simulink model "TestCase2_system_mapping"  (R2016a)
settings: Solver=FixedStepAuto  StartTime=0.0  StopTime=10.0  RelTol=1e-3
model workspace: external: MAT-File TestCase2_system_mapping.mat (data not in the file)
undefined symbols (not defined in the file or in its folder): obstacle
libraries: libTLAsserts x6, libAsserts x2
settings Model: Creator=Josef  LastModifiedBy=Josef
settings HardwareCC: ProdBitPerPointer=32  ProdWordSize=32  ProdHWDeviceType=Intel->x86-32 (Windows32)
settings GRTTargetCC: GeneratePreprocessorConditionals=Use local settings

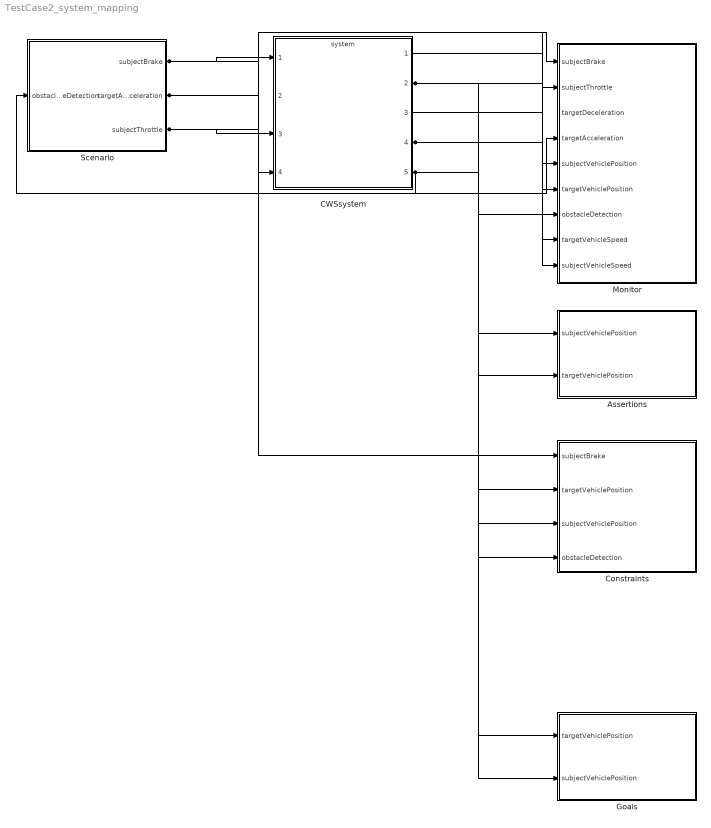
== system TestCase2_system_mapping ==
  Assertions : Subsystem
  CWSsystem : ModelReference  ModelNameDialog=system  SimulationMode=Normal  ModelReferenceVersion=1.18
  Constraints : Subsystem
  Goals : Subsystem
  Monitor : Subsystem
  Scenario : Subsystem
  wires:
  Scenario/3(subjectThrottle) -> CWSsystem/3, Monitor/2(subjectThrottle)
  Scenario/1(subjectBrake) -> CWSsystem/1, Monitor/1(subjectBrake), Constraints/1(subjectBrake)
  Scenario/2(targetAcceleration) -> CWSsystem/4, Monitor/4(targetAcceleration)
  CWSsystem/5 -> Scenario/1(obstacleDetection), Monitor/7(obstacleDetection), Constraints/4(obstacleDetection)
  CWSsystem/2 -> Monitor/5(subjectVehiclePosition), Assertions/1(subjectVehiclePosition), Constraints/3(subjectVehiclePosition), Goals/2(subjectVehiclePosition)
  CWSsystem/4 -> Monitor/6(targetVehiclePosition), Assertions/2(targetVehiclePosition), Constraints/2(targetVehiclePosition), Goals/1(targetVehiclePosition)
  CWSsystem/3 -> Monitor/8(targetVehicleSpeed)
  CWSsystem/1 -> Monitor/9(subjectVehicleSpeed)

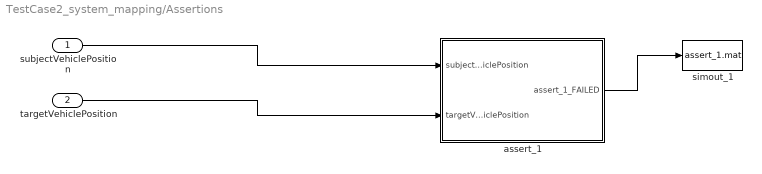
== system TestCase2_system_mapping/Assertions ==
  subjectVehiclePosition : Inport
  targetVehiclePosition : Inport  Port=2
  assert_1 : Subsystem
  simout_1 : ToFile  Filename=assert_1.mat  MatrixName=assert_1  SaveFormat=Timeseries
  wires:
  subjectVehiclePosition/1 -> assert_1/1(subjectVehiclePosition)
  targetVehiclePosition/1 -> assert_1/2(targetVehiclePosition)
  assert_1/1(assert_1_FAILED) -> simout_1/1

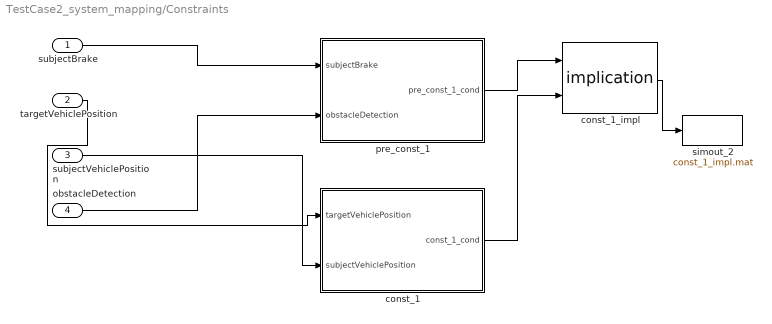
== system TestCase2_system_mapping/Constraints ==
  subjectBrake : Inport
  targetVehiclePosition : Inport  Port=2
  subjectVehiclePosition : Inport  Port=3
  obstacleDetection : Inport  Port=4
  const_1 : Subsystem
  const_1_impl : libAsserts/implication
  pre_const_1 : Subsystem
  simout_2 : ToFile  Filename=const_1_impl.mat  MatrixName=const_1_impl  SaveFormat=Timeseries
  wires:
  subjectBrake/1 -> pre_const_1/1(subjectBrake)
  obstacleDetection/1 -> pre_const_1/2(obstacleDetection)
  targetVehiclePosition/1 -> const_1/1(targetVehiclePosition)
  subjectVehiclePosition/1 -> const_1/2(subjectVehiclePosition)
  pre_const_1/1(pre_const_1_cond) -> const_1_impl/1
  const_1/1(const_1_cond) -> const_1_impl/2
  const_1_impl/1 -> simout_2/1

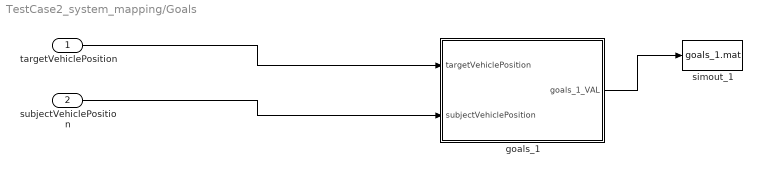
== system TestCase2_system_mapping/Goals ==
  targetVehiclePosition : Inport
  subjectVehiclePosition : Inport  Port=2
  goals_1 : Subsystem
  simout_1 : ToFile  Filename=goals_1.mat  MatrixName=goals_1  SaveFormat=Timeseries
  wires:
  targetVehiclePosition/1 -> goals_1/1(targetVehiclePosition)
  subjectVehiclePosition/1 -> goals_1/2(subjectVehiclePosition)
  goals_1/1(goals_1_VAL) -> simout_1/1

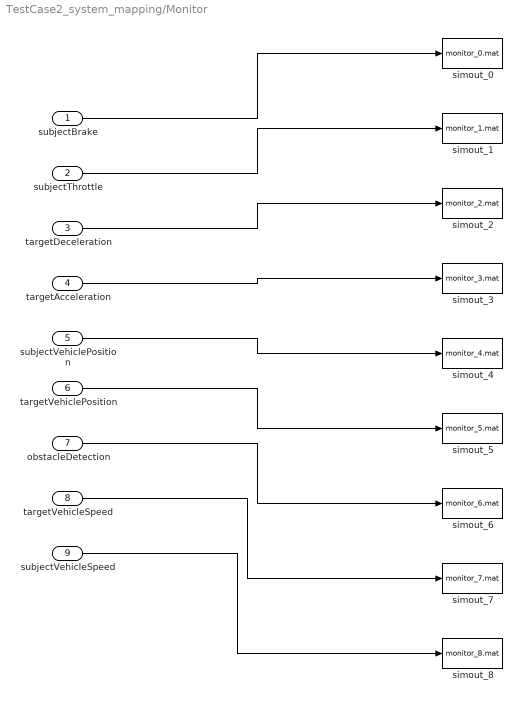
== system TestCase2_system_mapping/Monitor ==
  subjectBrake : Inport
  subjectThrottle : Inport  Port=2
  targetDeceleration : Inport  Port=3
  targetAcceleration : Inport  Port=4
  subjectVehiclePosition : Inport  Port=5
  targetVehiclePosition : Inport  Port=6
  obstacleDetection : Inport  Port=7
  targetVehicleSpeed : Inport  Port=8
  subjectVehicleSpeed : Inport  Port=9
  simout_0 : ToFile  Filename=monitor_0.mat  MatrixName=subjectBrake  SaveFormat=Timeseries
  simout_1 : ToFile  Filename=monitor_1.mat  MatrixName=subjectThrottle  SaveFormat=Timeseries
  simout_2 : ToFile  Filename=monitor_2.mat  MatrixName=targetDeceleration  SaveFormat=Timeseries
  simout_3 : ToFile  Filename=monitor_3.mat  MatrixName=targetAcceleration  SaveFormat=Timeseries
  simout_4 : ToFile  Filename=monitor_4.mat  MatrixName=subjectVehiclePosition  SaveFormat=Timeseries
  simout_5 : ToFile  Filename=monitor_5.mat  MatrixName=targetVehiclePosition  SaveFormat=Timeseries
  simout_6 : ToFile  Filename=monitor_6.mat  MatrixName=obstacleDetection  SaveFormat=Timeseries
  simout_7 : ToFile  Filename=monitor_7.mat  MatrixName=targetVehicleSpeed  SaveFormat=Timeseries
  simout_8 : ToFile  Filename=monitor_8.mat  MatrixName=subjectVehicleSpeed  SaveFormat=Timeseries
  wires:
  subjectBrake/1 -> simout_0/1
  subjectThrottle/1 -> simout_1/1
  targetDeceleration/1 -> simout_2/1
  targetAcceleration/1 -> simout_3/1
  subjectVehiclePosition/1 -> simout_4/1
  targetVehiclePosition/1 -> simout_5/1
  obstacleDetection/1 -> simout_6/1
  targetVehicleSpeed/1 -> simout_7/1
  subjectVehicleSpeed/1 -> simout_8/1

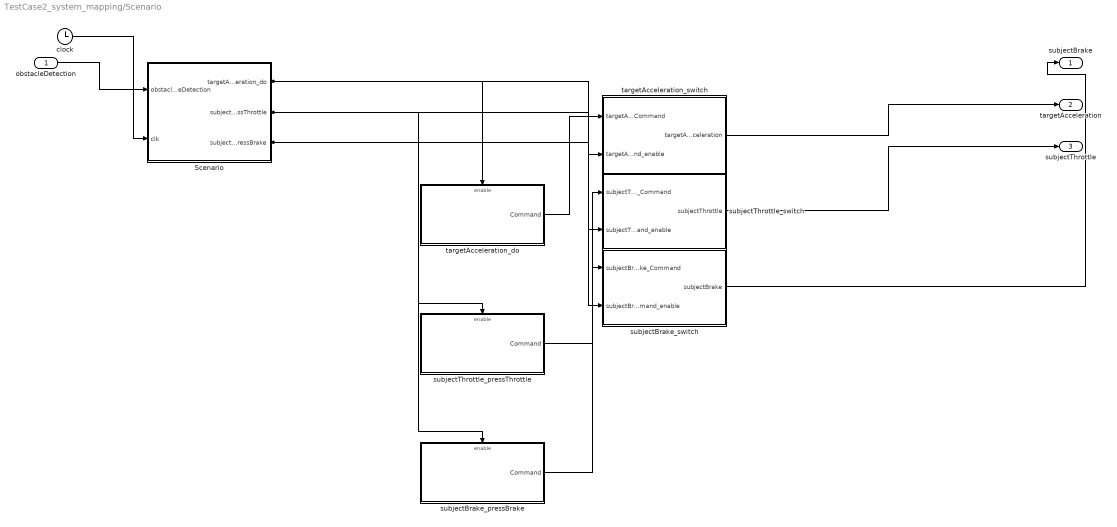
== system TestCase2_system_mapping/Scenario ==
  obstacleDetection : Inport
  Scenario : Stateflow chart  TreatAsAtomicUnit=on
  clock : Clock
  subjectBrake_pressBrake : Subsystem
  subjectBrake_switch : Subsystem
  subjectThrottle_pressThrottle : Subsystem
  subjectThrottle_switch : Subsystem
  targetAcceleration_do : Subsystem
  targetAcceleration_switch : Subsystem
  subjectBrake : Outport
  targetAcceleration : Outport  Port=2
  subjectThrottle : Outport  Port=3
  wires:
  targetAcceleration_switch/1(targetAcceleration) -> targetAcceleration/1
  subjectThrottle_switch/1(subjectThrottle) -> subjectThrottle/1
  subjectBrake_switch/1(subjectBrake) -> subjectBrake/1
  targetAcceleration_do/1(Command) -> targetAcceleration_switch/1(targetAcceleration_do_Command)
  Scenario/1(targetAcceleration_do) -> targetAcceleration_switch/2(targetAcceleration_do_Command_enable), targetAcceleration_do/Enable
  subjectThrottle_pressThrottle/1(Command) -> subjectThrottle_switch/1(subjectThrottle_pressThrottle_Command)
  Scenario/2(subjectThrottle_pressThrottle) -> subjectThrottle_switch/2(subjectThrottle_pressThrottle_Command_enable), subjectThrottle_pressThrottle/Enable
  subjectBrake_pressBrake/1(Command) -> subjectBrake_switch/1(subjectBrake_pressBrake_Command)
  Scenario/3(subjectBrake_pressBrake) -> subjectBrake_switch/2(subjectBrake_pressBrake_Command_enable), subjectBrake_pressBrake/Enable
  obstacleDetection/1 -> Scenario/1(obstacleDetection)
  clock/1 -> Scenario/2(clk)

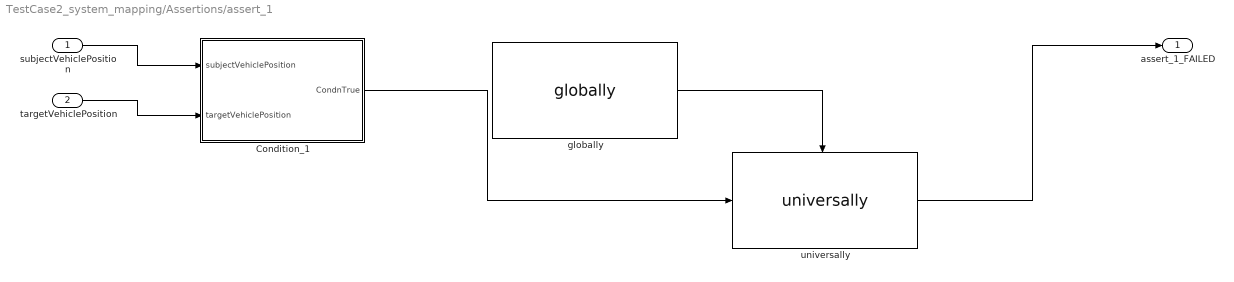
== system TestCase2_system_mapping/Assertions/assert_1 ==
  subjectVehiclePosition : Inport
  targetVehiclePosition : Inport  Port=2
  Condition_1 : Subsystem
  globally : libTLAsserts/globally
  universally : libTLAsserts/universally
  assert_1_FAILED : Outport
  wires:
  subjectVehiclePosition/1 -> Condition_1/1(subjectVehiclePosition)
  targetVehiclePosition/1 -> Condition_1/2(targetVehiclePosition)
  Condition_1/1(CondnTrue) -> universally/1
  globally/1 -> universally/Enable
  universally/1 -> assert_1_FAILED/1

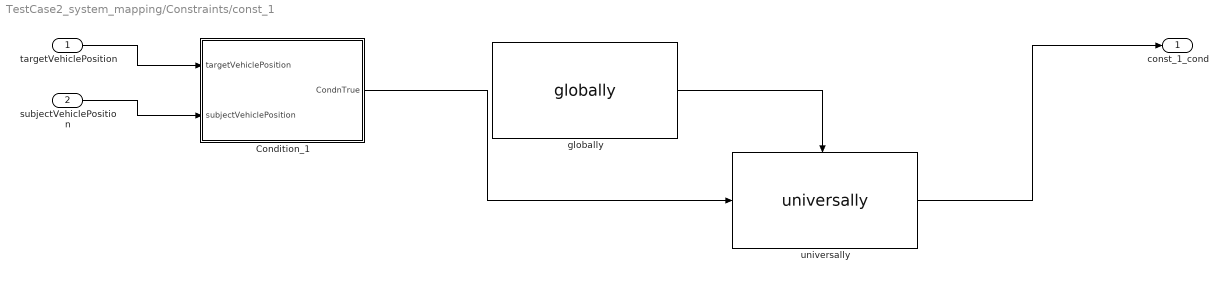
== system TestCase2_system_mapping/Constraints/const_1 ==
  targetVehiclePosition : Inport
  subjectVehiclePosition : Inport  Port=2
  Condition_1 : Subsystem
  globally : libTLAsserts/globally
  universally : libTLAsserts/universally
  const_1_cond : Outport
  wires:
  targetVehiclePosition/1 -> Condition_1/1(targetVehiclePosition)
  subjectVehiclePosition/1 -> Condition_1/2(subjectVehiclePosition)
  Condition_1/1(CondnTrue) -> universally/1
  globally/1 -> universally/Enable
  universally/1 -> const_1_cond/1

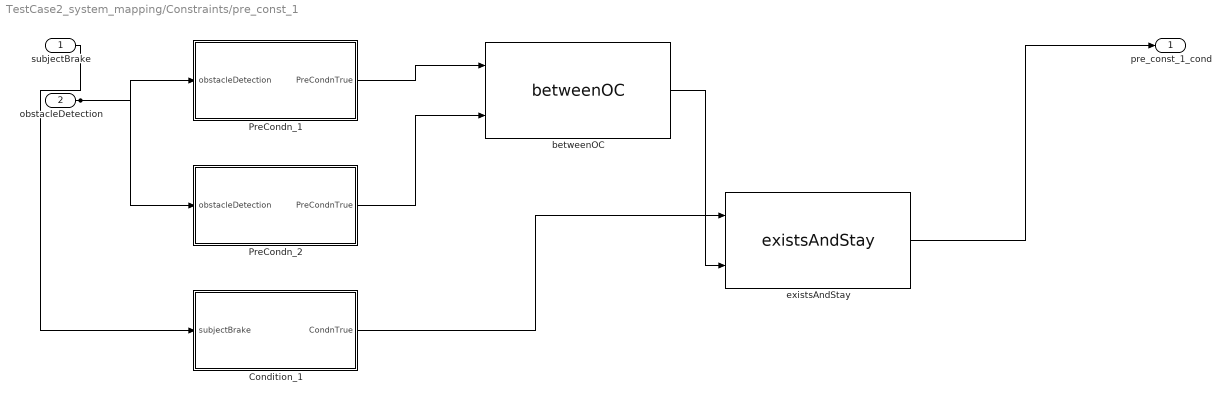
== system TestCase2_system_mapping/Constraints/pre_const_1 ==
  subjectBrake : Inport
  obstacleDetection : Inport  Port=2
  Condition_1 : Subsystem
  PreCondn_1 : Subsystem
  PreCondn_2 : Subsystem
  betweenOC : libTLAsserts/betweenOC
  existsAndStay : libTLAsserts/existsAndStay
  pre_const_1_cond : Outport
  wires:
  obstacleDetection/1 -> PreCondn_1/1(obstacleDetection), PreCondn_2/1(obstacleDetection)
  subjectBrake/1 -> Condition_1/1(subjectBrake)
  PreCondn_1/1(PreCondnTrue) -> betweenOC/1
  PreCondn_2/1(PreCondnTrue) -> betweenOC/2
  Condition_1/1(CondnTrue) -> existsAndStay/1
  betweenOC/1 -> existsAndStay/2
  existsAndStay/1 -> pre_const_1_cond/1

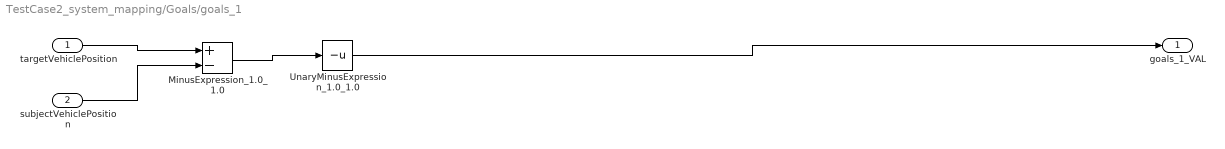
== system TestCase2_system_mapping/Goals/goals_1 ==
  targetVehiclePosition : Inport
  subjectVehiclePosition : Inport  Port=2
  MinusExpression_1.0_1.0 : Sum  Inputs=+-
  UnaryMinusExpression_1.0_1.0 : UnaryMinus
  goals_1_VAL : Outport
  wires:
  targetVehiclePosition/1 -> MinusExpression_1.0_1.0/1
  subjectVehiclePosition/1 -> MinusExpression_1.0_1.0/2
  MinusExpression_1.0_1.0/1 -> UnaryMinusExpression_1.0_1.0/1
  UnaryMinusExpression_1.0_1.0/1 -> goals_1_VAL/1

== system TestCase2_system_mapping/Scenario/subjectBrake_pressBrake ==
  Enable : EnablePort
  PedalPressed : Constant
  Command : Outport  OutputWhenDisabled=reset  InitialOutput=0
  wires:
  PedalPressed/1 -> Command/1

== system TestCase2_system_mapping/Scenario/subjectBrake_switch ==
  subjectBrake_pressBrake_Command : Inport
  subjectBrake_pressBrake_Command_enable : Inport  Port=2
  subjectBrake_pressBrake_Command_terminator : Terminator
  subjectBrake : Outport
  wires:
  subjectBrake_pressBrake_Command_enable/1 -> subjectBrake_pressBrake_Command_terminator/1
  subjectBrake_pressBrake_Command/1 -> subjectBrake/1

== system TestCase2_system_mapping/Scenario/subjectThrottle_pressThrottle ==
  Enable : EnablePort
  PedalPressed : Constant
  Command : Outport  OutputWhenDisabled=reset  InitialOutput=0
  wires:
  PedalPressed/1 -> Command/1

== system TestCase2_system_mapping/Scenario/subjectThrottle_switch ==
  subjectThrottle_pressThrottle_Command : Inport
  subjectThrottle_pressThrottle_Command_enable : Inport  Port=2
  subjectThrottle_pressThrottle_Command_terminator : Terminator
  subjectThrottle : Outport
  wires:
  subjectThrottle_pressThrottle_Command_enable/1 -> subjectThrottle_pressThrottle_Command_terminator/1
  subjectThrottle_pressThrottle_Command/1 -> subjectThrottle/1

== system TestCase2_system_mapping/Scenario/targetAcceleration_do ==
  Enable : EnablePort
  PedalPressed : Constant
  Command : Outport  OutputWhenDisabled=reset  InitialOutput=0
  wires:
  PedalPressed/1 -> Command/1

== system TestCase2_system_mapping/Scenario/targetAcceleration_switch ==
  targetAcceleration_do_Command : Inport
  targetAcceleration_do_Command_enable : Inport  Port=2
  targetAcceleration_do_Command_terminator : Terminator
  targetAcceleration : Outport
  wires:
  targetAcceleration_do_Command_enable/1 -> targetAcceleration_do_Command_terminator/1
  targetAcceleration_do_Command/1 -> targetAcceleration/1

== system TestCase2_system_mapping/Assertions/assert_1/Condition_1 ==
  subjectVehiclePosition : Inport
  targetVehiclePosition : Inport  Port=2
  GreaterExpression_1.0_1.0 : RelationalOperator  Operator=>  OutDataTypeStr=boolean
  CondnTrue : Outport
  wires:
  targetVehiclePosition/1 -> GreaterExpression_1.0_1.0/1
  subjectVehiclePosition/1 -> GreaterExpression_1.0_1.0/2
  GreaterExpression_1.0_1.0/1 -> CondnTrue/1

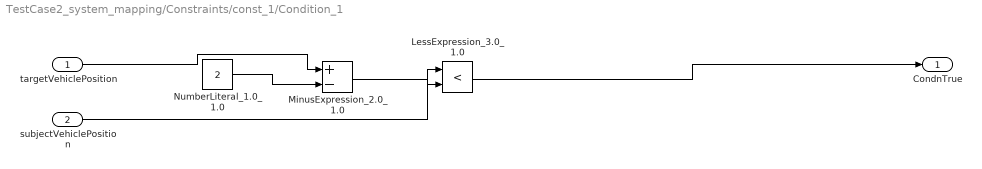
== system TestCase2_system_mapping/Constraints/const_1/Condition_1 ==
  targetVehiclePosition : Inport
  subjectVehiclePosition : Inport  Port=2
  LessExpression_3.0_1.0 : RelationalOperator  Operator=<  OutDataTypeStr=boolean
  MinusExpression_2.0_1.0 : Sum  Inputs=+-
  NumberLiteral_1.0_1.0 : Constant  Value=2
  CondnTrue : Outport
  wires:
  targetVehiclePosition/1 -> MinusExpression_2.0_1.0/1
  NumberLiteral_1.0_1.0/1 -> MinusExpression_2.0_1.0/2
  subjectVehiclePosition/1 -> LessExpression_3.0_1.0/1
  MinusExpression_2.0_1.0/1 -> LessExpression_3.0_1.0/2
  LessExpression_3.0_1.0/1 -> CondnTrue/1

== system TestCase2_system_mapping/Constraints/pre_const_1/Condition_1 ==
  subjectBrake : Inport
  EqualsExpression_2.0_1.0 : RelationalOperator  Operator===  OutDataTypeStr=boolean
  StringLiteral_1.0_1.0 : Constant
  CondnTrue : Outport
  wires:
  subjectBrake/1 -> EqualsExpression_2.0_1.0/1
  StringLiteral_1.0_1.0/1 -> EqualsExpression_2.0_1.0/2
  EqualsExpression_2.0_1.0/1 -> CondnTrue/1

== system TestCase2_system_mapping/Constraints/pre_const_1/PreCondn_1 ==
  obstacleDetection : Inport
  EqualsExpression_2.0_1.0 : RelationalOperator  Operator===  OutDataTypeStr=boolean
  StringLiteral_1.0_1.0 : Constant  Value=obstacle
  PreCondnTrue : Outport
  wires:
  obstacleDetection/1 -> EqualsExpression_2.0_1.0/1
  StringLiteral_1.0_1.0/1 -> EqualsExpression_2.0_1.0/2
  EqualsExpression_2.0_1.0/1 -> PreCondnTrue/1

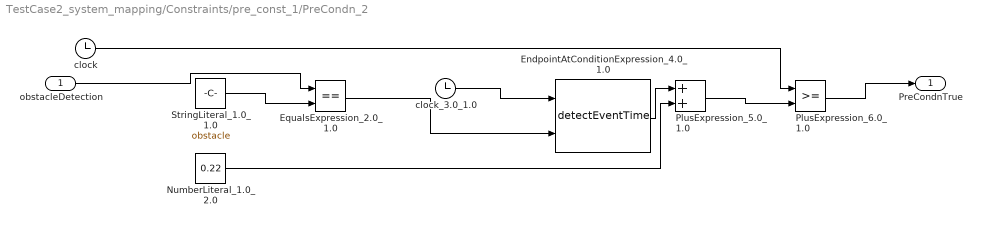
== system TestCase2_system_mapping/Constraints/pre_const_1/PreCondn_2 ==
  obstacleDetection : Inport
  EndpointAtConditionExpression_4.0_1.0 : libAsserts/detectEventTime
  EqualsExpression_2.0_1.0 : RelationalOperator  Operator===  OutDataTypeStr=boolean
  NumberLiteral_1.0_2.0 : Constant  Value=0.22
  PlusExpression_5.0_1.0 : Sum
  PlusExpression_6.0_1.0 : RelationalOperator  OutDataTypeStr=boolean
  StringLiteral_1.0_1.0 : Constant  Value=obstacle
  clock : Clock
  clock_3.0_1.0 : Clock
  PreCondnTrue : Outport
  wires:
  obstacleDetection/1 -> EqualsExpression_2.0_1.0/1
  StringLiteral_1.0_1.0/1 -> EqualsExpression_2.0_1.0/2
  clock_3.0_1.0/1 -> EndpointAtConditionExpression_4.0_1.0/1
  EqualsExpression_2.0_1.0/1 -> EndpointAtConditionExpression_4.0_1.0/2
  EndpointAtConditionExpression_4.0_1.0/1 -> PlusExpression_5.0_1.0/1
  NumberLiteral_1.0_2.0/1 -> PlusExpression_5.0_1.0/2
  clock/1 -> PlusExpression_6.0_1.0/1
  PlusExpression_5.0_1.0/1 -> PlusExpression_6.0_1.0/2
  PlusExpression_6.0_1.0/1 -> PreCondnTrue/1

== stateflow chart TestCase2_system_mapping/Scenario/Scenario ==
  state Act_Subject [parallel]
    settings: executionOrder=1
    state Act_Subject_Step1
      entry: subjectThrottle_pressThrottle = 1;
    state Act_Subject_Step2
      entry: Act_Subject_Step2_stpClk = clk;
    state Act_Subject_Step3
      entry: subjectThrottle_pressThrottle = 0;
      entry: subjectBrake_pressBrake = 1;
    (default) -> Act_Subject_Step1
    Act_Subject_Step1 -> Act_Subject_Step2 : [obstacleDetection]
    Act_Subject_Step2 -> Act_Subject_Step3 : [clk - Act_Subject_Step2_stpClk > 0.21]
  state Act_Target [parallel]
    settings: executionOrder=2
    state Act_Target_Step1
      entry: targetAcceleration_do = 1;
    state Act_Target_Step2
      entry: targetAcceleration_do = 0;
    (default) -> Act_Target_Step1
    Act_Target_Step1 -> Act_Target_Step2 : [clk > 10]
  data: obstacleDetection input; clk input; targetAcceleration_do output; subjectThrottle_pressThrottle output; subjectBrake_pressBrake output; Act_Subject_Step2_stpClk local
